simulink model "Task3_1"  (R2020b)
settings: Solver=VariableStepAuto  StartTime=0.0  StopTime=100.0  RelTol=1e-3
values from neighbouring files (symbols this model uses):
  a1 = c0 * pi * rho * r^3    (= 10823.7684393)    [Code2021_Jo_Saleh.m]    (also in ExeRet21.m.m)
  a2 = c1 * pi * rho * r^4 / p    (= 2913.06360466)    [Code2021_Jo_Saleh.m]    (also in ExeRet21.m.m)
  a3 = 4 * c2 * pi * rho * r^5 / p^2    (= -341.490636632)    [Code2021_Jo_Saleh.m]    (also in ExeRet21.m.m)
  D = 0    [Code2021_Jo_Saleh.m]    (also in ExeRet21.m.m)
  dTe = 1e5    (= 100000)    [Code2021_Jo_Saleh.m]    (also in ExeRet21.m.m)
  dVw = 0.1    [Code2021_Jo_Saleh.m]    (also in ExeRet21.m.m)
  J = H * 2 * Sb / wm^2    (= 9574851.8542)    [Code2021_Jo_Saleh.m]    (also in ExeRet21.m.m)
  p = 180    [Code2021_Jo_Saleh.m]    (also in ExeRet21.m.m)
  tau_w = - 2 * J / (p * (a2*Vw_3 + a3*we_opt - D*2/p))    (= 8.82652066845)    [Code2021_Jo_Saleh.m]    (also in ExeRet21.m.m)
  tau_z = tau_w / (1 - p * tau_w * Te_opt / (2 * we_opt * J))    (= -109.330180381)    [Code2021_Jo_Saleh.m]    (also in ExeRet21.m.m)
  Te_rated = (Ptur * p) / (2 * we)    (= 1671126.90246)    [Code2021_Jo_Saleh.m]    (also in ExeRet21.m.m)
  Vw_3 = 10    [Code2021_Jo_Saleh.m]    (also in ExeRet21.m.m)
  we_opt = p / 2 * wm_opt    (= 120.6)    [Code2021_Jo_Saleh.m]    (also in ExeRet21.m.m)
settings Model: Creator=Tomo  LastModifiedBy=Tomo

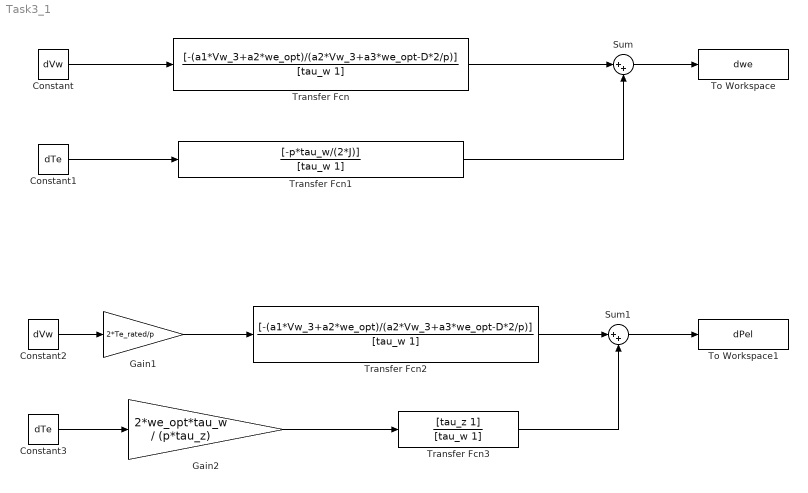
== system Task3_1 ==
  Constant : Constant  Value=dVw
  Constant1 : Constant  Value=dTe
  Constant2 : Constant  Value=dVw
  Constant3 : Constant  Value=dTe
  Gain1 : Gain  Gain=2*Te_rated/p
  Gain2 : Gain  Gain=2*we_opt*tau_w / (p*tau_z)
  Sum : Sum  Inputs=|++
  Sum1 : Sum  Inputs=|++
  To Workspace : ToWorkspace  VariableName=dwe  SampleTime=-1
  To Workspace1 : ToWorkspace  VariableName=dPel  SampleTime=-1
  Transfer Fcn : TransferFcn  Numerator=[-(a1*Vw_3+a2*we_opt)/(a2*Vw_3+a3*we_opt-D*2/p)]  Denominator=[tau_w 1]
  Transfer Fcn1 : TransferFcn  Numerator=[-p*tau_w/(2*J)]  Denominator=[tau_w 1]
  Transfer Fcn2 : TransferFcn  Numerator=[-(a1*Vw_3+a2*we_opt)/(a2*Vw_3+a3*we_opt-D*2/p)]  Denominator=[tau_w 1]
  Transfer Fcn3 : TransferFcn  Numerator=[tau_z 1]  Denominator=[tau_w 1]
  wires:
  Constant/1 -> Transfer Fcn/1
  Transfer Fcn/1 -> Sum/1
  Transfer Fcn1/1 -> Sum/2
  Sum/1 -> To Workspace/1
  Gain1/1 -> Transfer Fcn2/1
  Constant2/1 -> Gain1/1
  Sum1/1 -> To Workspace1/1
  Transfer Fcn3/1 -> Sum1/2
  Gain2/1 -> Transfer Fcn3/1
  Constant3/1 -> Gain2/1
  Transfer Fcn2/1 -> Sum1/1
  Constant1/1 -> Transfer Fcn1/1
